simulink subsystem "Power_Limit"  (R2021b)
settings: Solver=VariableStepAuto  StartTime=0.0  StopTime=10.0  RelTol=1e-3
settings Model: Creator=tsuyoshi  LastModifiedBy=FEM

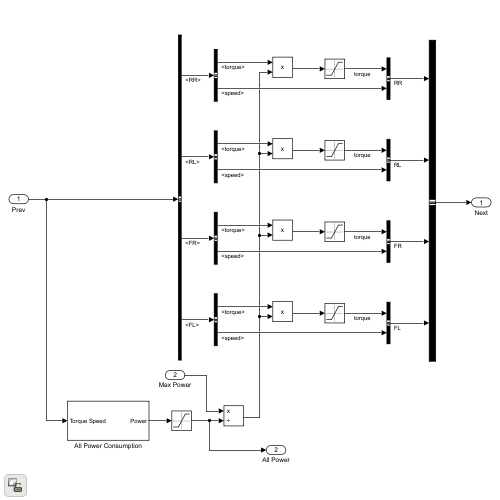
[thumbnail: Simulink's stored preview of the top-level diagram]
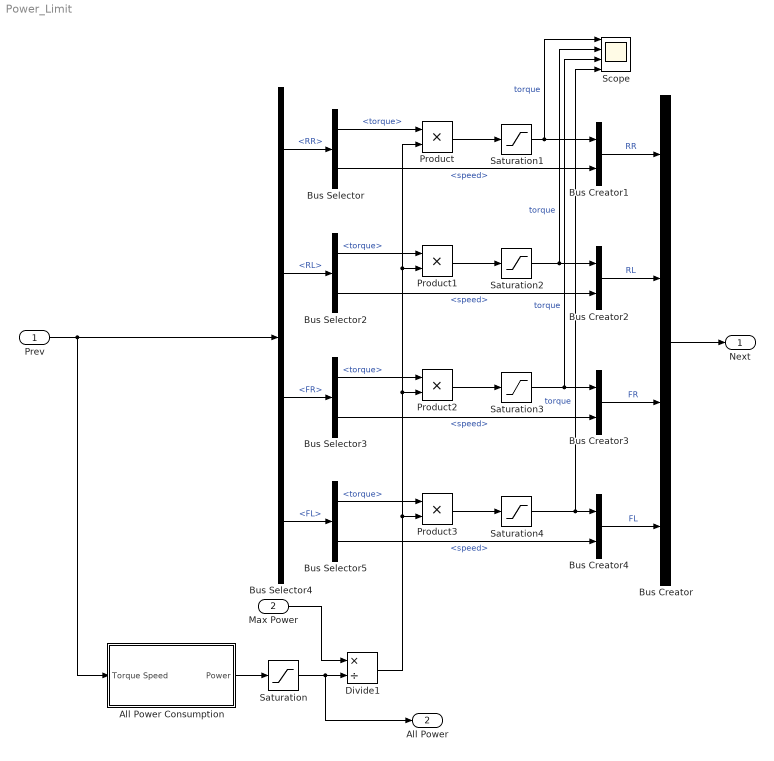
== system Power_Limit ==
  Prev : Inport
  Max Power : Inport  Port=2
  All Power Consumption : Subsystem
  Bus Creator : BusCreator  Inputs=4
  Bus Creator{1..4} (4 alike) : BusCreator  Inputs=2
  Bus Selector{,2..3,5} (4 alike) : BusSelector  OutputSignals=torque,speed
  Bus Selector4 : BusSelector  OutputSignals=RR,RL,FR,FL
  Divide1 : Product  Inputs=*/
  Product{,1..3} (4 alike) : Product
  Saturation : Saturate  UpperLimit=inf  LowerLimit=1
  Saturation{1..4} (4 alike) : Saturate  UpperLimit=21  LowerLimit=-21
  Scope : Scope  NumInputPorts=4
  Next : Outport  VectorParamsAs1DForOutWhenUnconnected=off
  All Power : Outport  Port=2  VectorParamsAs1DForOutWhenUnconnected=off
  wires:
  Max Power/1 -> Divide1/1
  Bus Creator/1 -> Next/1
  Prev/1 -> Bus Selector4/1, All Power Consumption/1(Torque Speed)
  Bus Selector/2 -> Bus Creator1/2  "<speed>"
  Saturation/1 -> Divide1/2, All Power/1
  Bus Selector/1 -> Product/1  "<torque>"
  Product/1 -> Saturation1/1
  Bus Creator1/1 -> Bus Creator/1  "RR"
  Saturation1/1 -> Scope/1, Bus Creator1/1  "torque"
  Saturation2/1 -> Scope/2, Bus Creator2/1  "torque"
  Bus Creator2/1 -> Bus Creator/2  "RL"
  Product1/1 -> Saturation2/1
  Bus Selector2/1 -> Product1/1  "<torque>"
  Bus Selector2/2 -> Bus Creator2/2  "<speed>"
  Bus Selector3/2 -> Bus Creator3/2  "<speed>"
  Bus Selector3/1 -> Product2/1  "<torque>"
  Product2/1 -> Saturation3/1
  Bus Creator3/1 -> Bus Creator/3  "FR"
  Saturation3/1 -> Scope/3, Bus Creator3/1  "torque"
  Saturation4/1 -> Scope/4, Bus Creator4/1  "torque"
  Product3/1 -> Saturation4/1
  Bus Selector5/1 -> Product3/1  "<torque>"
  Bus Selector5/2 -> Bus Creator4/2  "<speed>"
  Bus Creator4/1 -> Bus Creator/4  "FL"
  Bus Selector4/1 -> Bus Selector/1  "<RR>"
  Bus Selector4/2 -> Bus Selector2/1  "<RL>"
  Bus Selector4/3 -> Bus Selector3/1  "<FR>"
  Bus Selector4/4 -> Bus Selector5/1  "<FL>"
  Divide1/1 -> Product2/2, Product/2, Product1/2, Product3/2
  All Power Consumption/1(Power) -> Saturation/1

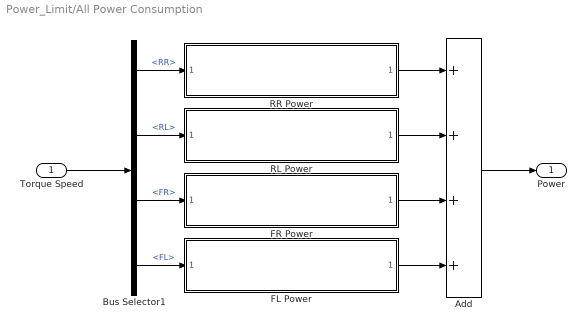
== system Power_Limit/All Power Consumption ==
  Torque Speed : Inport
  Add : Sum  Inputs=++++
  Bus Selector1 : BusSelector  OutputSignals=RR,RL,FR,FL
  FL Power : Subsystem  ReferencedSubsystem=OneMotorPower
  FR Power : Subsystem  ReferencedSubsystem=OneMotorPower
  RL Power : Subsystem  ReferencedSubsystem=OneMotorPower
  RR Power : Subsystem  ReferencedSubsystem=OneMotorPower
  Power : Outport
  wires:
  Torque Speed/1 -> Bus Selector1/1
  Add/1 -> Power/1
  Bus Selector1/4 -> FL Power/1  "<FL>"
  Bus Selector1/2 -> RL Power/1  "<RL>"
  FR Power/1 -> Add/3
  FL Power/1 -> Add/4
  Bus Selector1/3 -> FR Power/1  "<FR>"
  RR Power/1 -> Add/1
  Bus Selector1/1 -> RR Power/1  "<RR>"
  RL Power/1 -> Add/2
